simulink model "ModelLinearMechFram"  (R2014b)
settings: Solver=ode45  StartTime=0.0  StopTime=2  FixedStep=0.001  RelTol=1e-3
values from neighbouring files (symbols this model uses):
  H1 = -(R4*Rs/R1) * 1/(R7+Rv2)    [InitModel.m]    (also in SystemModel.m)
  R6 = 100e3    (= 100000)    [InitModel.m]    (also in SystemModel.m; SystemModel_marco.m)
  rad2rpm = 60/(2*pi)    (= 9.54929658551)    [InitModel.m]    (also in SystemModel.m)
  Vdc = 30    [InitModel.m]    (also in SystemModel.m; SystemModel_marco.m)
undefined symbols (not defined in the file or in its folder): motor
libraries: cstblocks x7, simulink x1
settings Model: Creator=Edoardo  LastModifiedBy=marco

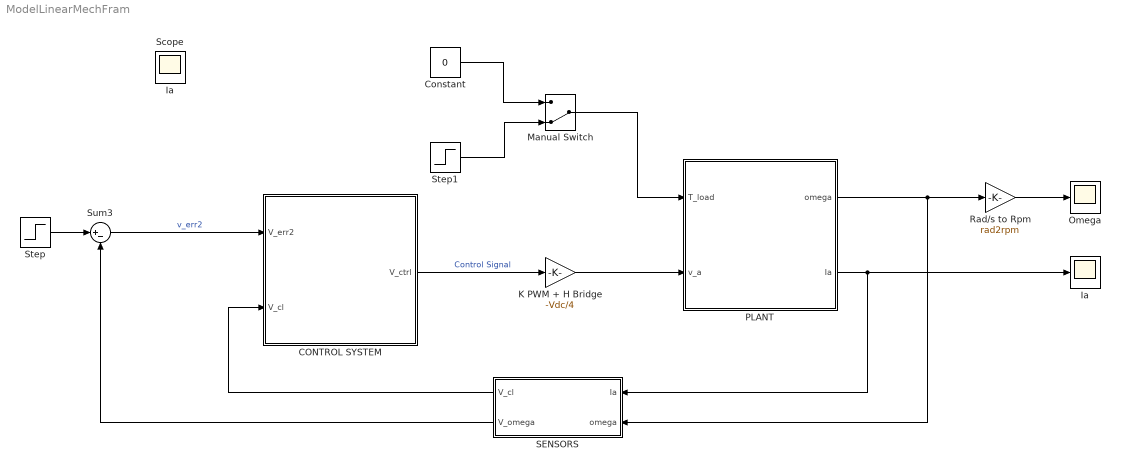
== system ModelLinearMechFram ==
  CONTROL SYSTEM : Subsystem
  Constant : Constant  Value=0
  "Ia " : Scope
      settings: YMin=-0.2  YMax=1.4  SaveName=ScopeData3
  K PWM + H Bridge : Gain  Gain=-Vdc/4
  Manual Switch : ManualSwitch  CurrentSetting=0
  Omega : Scope
      settings: TimeRange=2  YMin=-25000  YMax=5000
  PLANT : Subsystem
  Rad/s to Rpm : Gain  Gain=rad2rpm
  SENSORS : Subsystem
  Step : Step  Time=0  After=4  SampleTime=0
  Step1 : Step  Time=0.1  After=0.06
  Sum3 : Sum  Inputs=|+-
  Ia : Scope
  Scope : Scope
      settings: YMin=-2  YMax=12  SaveName=ScopeData2  Decimation=10
  wires:
  Rad/s to Rpm/1 -> Omega/1
  Step/1 -> Sum3/1
  K PWM + H Bridge/1 -> PLANT/2(v_a)
  PLANT/1(omega) -> SENSORS/2(omega), Rad/s to Rpm/1
  Sum3/1 -> CONTROL SYSTEM/1(V_err2)  "v_err2"
  CONTROL SYSTEM/1(V_ctrl) -> K PWM + H Bridge/1  "Control Signal"
  PLANT/2(Ia) -> SENSORS/1(Ia), "Ia "/1
  SENSORS/2(V_omega) -> Sum3/2
  SENSORS/1("V_cl ") -> CONTROL SYSTEM/2(V_cl)
  Manual Switch/1 -> PLANT/1(T_load)
  Constant/1 -> Manual Switch/1
  Step1/1 -> Manual Switch/2

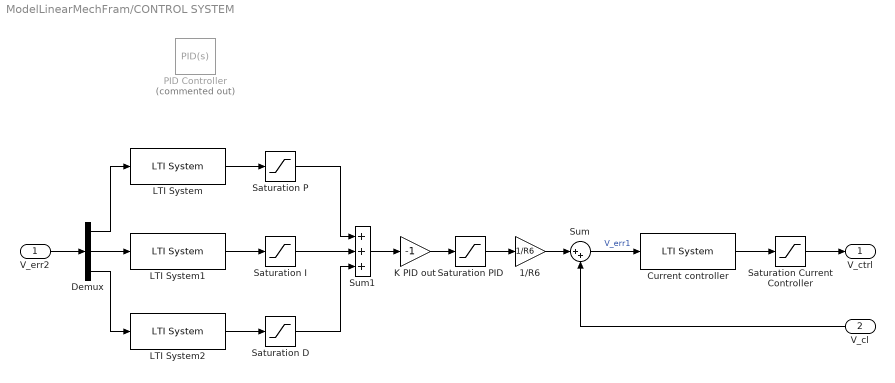
== system ModelLinearMechFram/CONTROL SYSTEM ==
  V_err2 : Inport
  V_cl : Inport  Port=2
  1/R6 : Gain  Gain=1/R6
  Current controller : cstblocks/LTI System  sys=C1  IC=[]
  Demux : Demux  Outputs=3
  K PID out : Gain  Gain=-1
  LTI System : cstblocks/LTI System  sys=pid.p  IC=[]
  LTI System1 : cstblocks/LTI System  sys=pid.i  IC=[]
  LTI System2 : cstblocks/LTI System  sys=pid.d  IC=[]
  PID Controller : simulink/Continuous/PID Controller  Commented=on  Controller=PID  TimeDomain=Continuous-time  SampleTime=-1  IntegratorMethod=Forward Euler  FilterMethod=Forward Euler  Form=Parallel  P=-0.00231296581948099  I=-0.000145342228739108  D=0.0110285788862625  N=0.209724738185631  InitialConditionSource=internal  InitialConditionForIntegrator=0  InitialConditionForFilter=0  ExternalReset=none  LimitOutput=off  UpperSaturationLimit=12  LowerSaturationLimit=-12  LinearizeAsGain=on  AntiWindupMode=clamping  Kb=1  TrackingMode=off  Kt=1  PParamMin=[]  PParamMax=[]  IParamMin=[]  IParamMax=[]  DParamMin=[]  DParamMax=[]  NParamMin=[]  NParamMax=[]  KbParamMin=[]  KbParamMax=[]  KtParamMin=[]  KtParamMax=[]  POutMin=[]  POutMax=[]  IOutMin=[]  IOutMax=[]  DOutMin=[]  DOutMax=[]  NOutMin=[]  NOutMax=[]  KbOutMin=[]  KbOutMax=[]  KtOutMin=[]  KtOutMax=[]  IntegratorOutMin=[]  IntegratorOutMax=[]  FilterOutMin=[]  FilterOutMax=[]  SumOutMin=[]  SumOutMax=[]  SumI1OutMin=[]  SumI1OutMax=[]  SumI2OutMin=[]  SumI2OutMax=[]  SumI3OutMin=[]  SumI3OutMax=[]  SumDOutMin=[]  SumDOutMax=[]  SaturationOutMin=[]  SaturationOutMax=[]  IntegratorContinuousStateAttributes=''  IntegratorStateMustResolveToSignalObject=off  IntegratorRTWStateStorageClass=Auto  FilterContinuousStateAttributes=''  FilterStateMustResolveToSignalObject=off  FilterRTWStateStorageClass=Auto  DifferentiatorICPrevScaledInput=0  DifferentiatorOutMin=[]  DifferentiatorOutMax=[]  UseFilter=on
  Saturation Current Controller : Saturate  UpperLimit=12  LowerLimit=-12
  Saturation D : Saturate  UpperLimit=12  LowerLimit=-12
  Saturation I : Saturate  UpperLimit=12  LowerLimit=-12
  Saturation P : Saturate  UpperLimit=12  LowerLimit=-12
  Saturation PID : Saturate  UpperLimit=9.1  LowerLimit=-9.1
  Sum : Sum  Inputs=|++
  Sum1 : Sum  Inputs=+++
  V_ctrl : Outport
  wires:
  1/R6/1 -> Sum/1
  Current controller/1 -> Saturation Current Controller/1
  Sum/1 -> Current controller/1  "V_err1"
  V_cl/1 -> Sum/2
  Saturation Current Controller/1 -> V_ctrl/1
  Demux/2 -> LTI System1/1
  Demux/1 -> LTI System/1
  Demux/3 -> LTI System2/1
  LTI System1/1 -> Saturation I/1
  LTI System2/1 -> Saturation D/1
  LTI System/1 -> Saturation P/1
  Saturation I/1 -> Sum1/2
  Saturation P/1 -> Sum1/1
  Saturation D/1 -> Sum1/3
  Saturation PID/1 -> 1/R6/1
  K PID out/1 -> Saturation PID/1
  V_err2/1 -> Demux/1
  Sum1/1 -> K PID out/1

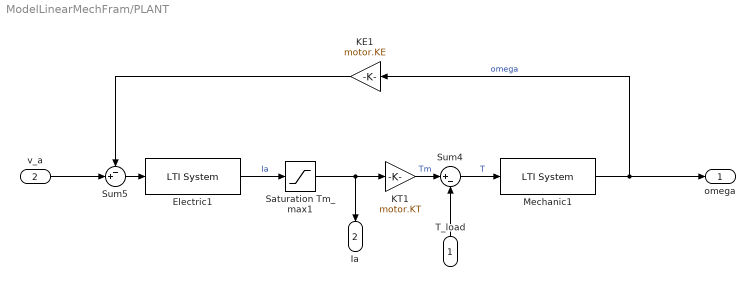
== system ModelLinearMechFram/PLANT ==
  T_load : Inport
  v_a : Inport  Port=2
  Electric1 : cstblocks/LTI System  sys=G1  IC=[]
  KE1 : Gain  Gain=motor.KE
  KT1 : Gain  Gain=motor.KT
  Mechanic1 : cstblocks/LTI System  sys=G2  IC=[]
  Saturation Tm_max1 : Saturate  UpperLimit=motor.Ia_max  LowerLimit=-motor.Ia_max
  Sum4 : Sum  Inputs=|+-
  Sum5 : Sum  Inputs=-+|
  omega : Outport
  Ia : Outport  Port=2
  wires:
  Electric1/1 -> Saturation Tm_max1/1  "Ia"
  KT1/1 -> Sum4/1  "Tm"
  Sum4/1 -> Mechanic1/1  "T"
  T_load/1 -> Sum4/2
  v_a/1 -> Sum5/2
  Sum5/1 -> Electric1/1
  Mechanic1/1 -> omega/1, KE1/1  "omega"
  KE1/1 -> Sum5/1
  Saturation Tm_max1/1 -> KT1/1, Ia/1

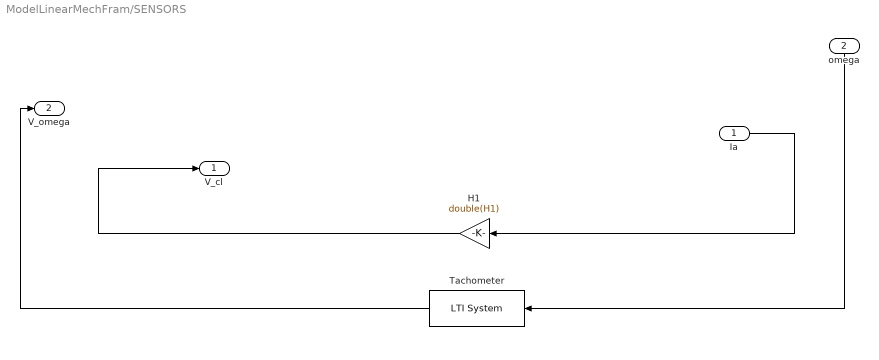
== system ModelLinearMechFram/SENSORS ==
  Ia : Inport
  omega : Inport  Port=2
  H1 : Gain  Gain=double(H1)
  Tachometer : cstblocks/LTI System  sys=H2  IC=[]
  "V_cl " : Outport
  V_omega : Outport  Port=2
  wires:
  Tachometer/1 -> V_omega/1
  H1/1 -> "V_cl "/1
  Ia/1 -> H1/1
  omega/1 -> Tachometer/1
